simulink model "old_style_sim_model"  (R2019b)
settings: Solver=VariableStepAuto  StartTime=0.0  StopTime=10.0  RelTol=1e-3
settings Model: Creator=njozw  LastModifiedBy=njozw

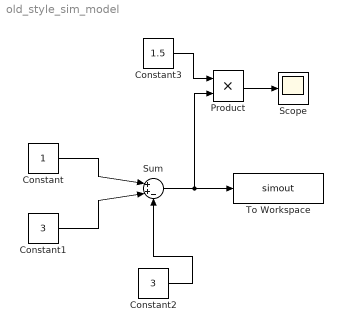
== system old_style_sim_model ==
  Constant : Constant
  Constant1 : Constant  Value=3
  Constant2 : Constant  Value=3
  Constant3 : Constant  Value=1.5
  Product : Product
  Scope : Scope
  Sum : Sum  Inputs=|++-
  To Workspace : ToWorkspace  VariableName=simout  SaveFormat=Timeseries  SampleTime=-1
  wires:
  Constant/1 -> Sum/1
  Constant1/1 -> Sum/2
  Sum/1 -> Product/2, To Workspace/1
  Constant2/1 -> Sum/3
  Product/1 -> Scope/1
  Constant3/1 -> Product/1
